simulink model "full_system_forDispatch_lut"  (R2015b)
settings: Solver=VariableStepAuto  StartTime=0.0  StopTime=7  FixedStep=1  RelTol=1e-2
values from neighbouring files (symbols this model uses):
  G1 = 12    [Parameters.m]
  G2 = 50    [Parameters.m]
  Kt = .07329    (= 0.07329)    [Parameters.m]
  L = 1e-4/2    (= 5e-05)    [Parameters.m]
  N = 4    [Parameters.m]
  r = 11*.0254/2    (= 0.1397)    [Parameters.m]
undefined symbols (not defined in the file or in its folder): ad, aq, bd, bq, c_drag_pro, cd, cq, DiscIntNeverNeededParam, dynamic, F_N, Ki, Kp, magnitude, n1, n2, sigbuilder_block, static, T, third_phase, viscous
libraries: fl_lib x24, nesl_utility x16, simulink x3, pe_lib x2
settings Model: Creator=Martin Andersen  LastModifiedBy=Martin Andersen
settings SolverCC: AlgebraicLoopSolver=LineSearch

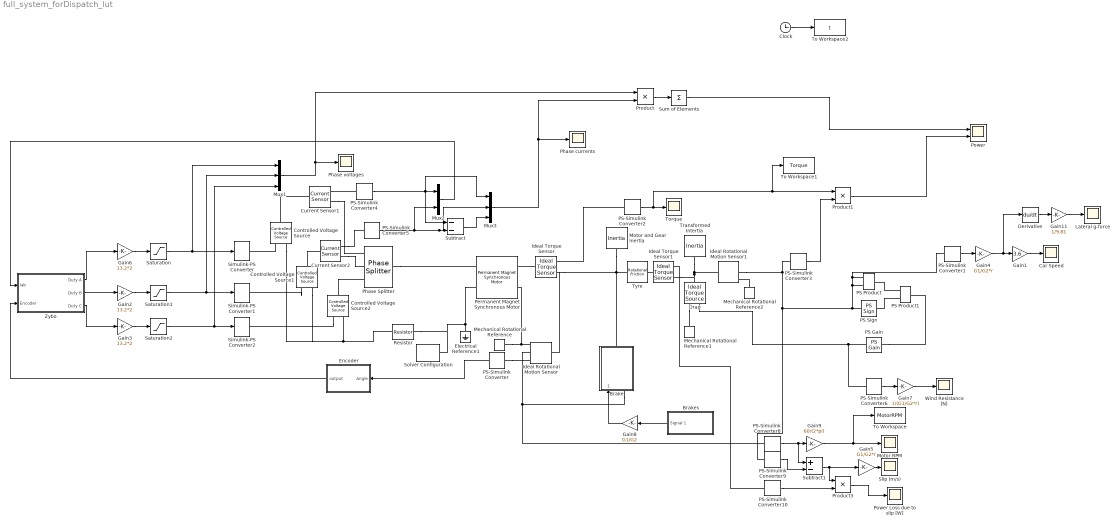
== system full_system_forDispatch_lut ==
  Brake : Subsystem
  Brakes : Subsystem  Tag=STV Subsys  LoadFcn=sigbuilder_block('load');  StartFcn=sigbuilder_block('start');  StopFcn=sigbuilder_block('stop');  ClipboardFcn=sigbuilder_block('clipboard');  mask(Sigbuilder block){}
      mask help: Simulink:masks:SigbuilderBlock_MD
      mask init:
      | if ~strcmp(get_param(bdroot(gcbh),'SimulationStatus'),'stopped') tuvar = sigbuilder_block('maskInit'); end
      settings: CopyFcn=sigbuilder_block('copy');  DeleteFcn=sigbuilder_block('delete');  ModelCloseFcn=sigbuilder_block('modelClose');  PreSaveFcn=sigbuilder_block('preSave');  PauseFcn=sigbuilder_block('pause');  ContinueFcn=sigbuilder_block('continue');  NameChangeFcn=sigbuilder_block('namechange');  OpenFcn=sigbuilder_block('open',[437.6 199.2 550.4 400 ]);  CloseFcn=sigbuilder_block('close');
      mask Display: plot(0, 0, 100, 100,[2, 2, 32, 32, 2], [68, 8, 8, 68, 68],[32, 2], [38, 38], [32, 19, 2],[53, 60, 44], [32, 17, 17, 2],[16, 16, 31, 31]);txt = getActiveGroup(gcbh);text(2, 100, txt,'verticalAlignment', 'top');
  Car Speed : Scope
  Clock : Clock
  Controlled Voltage Source : fl_lib/Electrical/Electrical Sources/Controlled Voltage Source
  Controlled Voltage Source1 : fl_lib/Electrical/Electrical Sources/Controlled Voltage Source
  Controlled Voltage Source2 : fl_lib/Electrical/Electrical Sources/Controlled Voltage Source
  Current Sensor1 : fl_lib/Electrical/Electrical Sensors/Current Sensor
  Current Sensor2 : fl_lib/Electrical/Electrical Sensors/Current Sensor
  Derivative : Derivative
  Drag : fl_lib/Mechanical/Mechanical Sources/Ideal Torque Source
  Electrical Reference1 : fl_lib/Electrical/Electrical Elements/Electrical Reference
  Encoder : Subsystem
  Gain1 : Gain  Gain=3.6
  Gain11 : Gain  Gain=1/9.81
  Gain2 : Gain  Gain=13.2*2
  Gain3 : Gain  Gain=13.2*2
  Gain4 : Gain  Gain=G1/G2*r
  Gain5 : Gain  Gain=G1/G2*r
  Gain6 : Gain  Gain=13.2*2
  Gain7 : Gain  Gain=1/(G1/G2*r)
  Gain8 : Gain  Gain=G1/G2
  Gain9 : Gain  Gain=60/(2*pi)
  Ideal Rotational Motion Sensor : fl_lib/Mechanical/Mechanical Sensors/Ideal Rotational Motion Sensor  offset=0 rad
  Ideal Rotational Motion Sensor1 : fl_lib/Mechanical/Mechanical Sensors/Ideal Rotational Motion Sensor  offset=0 rad
  Ideal Torque Sensor : fl_lib/Mechanical/Mechanical Sensors/Ideal Torque Sensor
  Ideal Torque Sensor1 : fl_lib/Mechanical/Mechanical Sensors/Ideal Torque Sensor
  Lateral g-force : Scope
  Mechanical Rotational Reference : fl_lib/Mechanical/Rotational Elements/Mechanical Rotational Reference
  Mechanical Rotational Reference1 : fl_lib/Mechanical/Rotational Elements/Mechanical Rotational Reference
  Mechanical Rotational Reference2 : fl_lib/Mechanical/Rotational Elements/Mechanical Rotational Reference
  Motor RPM : Scope
  Motor and Gear inertia : fl_lib/Mechanical/Rotational Elements/Inertia  inertia=J_pro1 kg*m^2  w_specify=off  w_priority=None  w=0 rad/s  t_specify=off  t_priority=None  t=0 N*m
  Mux1 : Mux  Inputs=3
  Mux2 : Mux  Inputs=2
  Mux3 : Mux  Inputs=3
  PS Gain : fl_lib/Physical Signals/Functions/PS Gain  gain=c_drag_pro
  PS Product : fl_lib/Physical Signals/Functions/PS Product
  PS Product1 : fl_lib/Physical Signals/Functions/PS Product
  PS Sign : fl_lib/Physical Signals/Nonlinear Operators/PS Sign
  PS-Simulink Converter{,1..6,8..10} (10 alike) : nesl_utility/PS-Simulink Converter  PhysicalDomain=network_engine_domain  SubClassName=ps_output  LeftPortType=input  RightPortType=output  PseudoPeriodic=off  Frequencies=[]  Unit=1  AffineConversion=off
  Permanent Magnet Synchronous Motor : pe_lib/Machines/Permanent Magnet Rotor/Permanent Magnet Synchronous Motor  nPolePairs=N  pm_flux_linkage=Kt/N Wb  stator_param=1  Ld=L H  Lq=L H  L0=L H  Ls=L H  Lm=0 H  Ms=L/10 H  Rs=R Ohm  initial_currents=[0, 0, 0] A  axes_param=2  angular_position0=0 rad  rotor_offset=- pi / 2 rad  shift_3ph=[nan, nan, nan] rad  sqrt2OverSqrt3=nan  oneOverSqrt2=nan  twoPiOver3=nan  Lmin=1e-9 H
  Phase Splitter : pe_lib/Connections/Phase Splitter
  Phase currents : Scope
  Phase voltages : Scope
  Power : Scope  NumInputPorts=2
  Power Loss due to slip [W] : Scope
  Product : Product
  Product1 : Product
  Product3 : Product
  Resistor : fl_lib/Electrical/Electrical Elements/Resistor  R=1e9 Ohm  i_specify=off  i_priority=None  i=0 A  v_specify=off  v_priority=None  v=0 V
  Saturation : Saturate  UpperLimit=13.2*2  LowerLimit=-13.2*2
  Saturation1 : Saturate  UpperLimit=13.2*2  LowerLimit=-13.2*2
  Saturation2 : Saturate  UpperLimit=13.2*2  LowerLimit=-13.2*2
  Simulink-PS Converter : nesl_utility/Simulink-PS Converter  PhysicalDomain=network_engine_domain  SubClassName=ps_input  LeftPortType=input  RightPortType=output  PseudoPeriodic=off  Frequencies=[]  NoiseDistribution=none  NoiseParameters=[]  Unit=1  AffineConversion=off  InputFiltering=off  SimscapeFilterOrder=1  InputFilterTimeConstant=0.001  UdotUserProvided=1
  Simulink-PS Converter1 : nesl_utility/Simulink-PS Converter  PhysicalDomain=network_engine_domain  SubClassName=ps_input  LeftPortType=input  RightPortType=output  PseudoPeriodic=off  Frequencies=[]  NoiseDistribution=none  NoiseParameters=[]  Unit=1  AffineConversion=off  InputFiltering=off  SimscapeFilterOrder=1  InputFilterTimeConstant=0.001  UdotUserProvided=1
  Simulink-PS Converter2 : nesl_utility/Simulink-PS Converter  PhysicalDomain=network_engine_domain  SubClassName=ps_input  LeftPortType=input  RightPortType=output  PseudoPeriodic=off  Frequencies=[]  NoiseDistribution=none  NoiseParameters=[]  Unit=1  AffineConversion=off  InputFiltering=off  SimscapeFilterOrder=1  InputFilterTimeConstant=0.001  UdotUserProvided=1
  Slip (m/s) : Scope
  Solver Configuration : nesl_utility/Solver Configuration  PhysicalDomain=network_engine_domain  SubClassName=solver  LeftPortType=input  RightPortType=generic  Accelerate=off  Tones=[]  Harmonics=[]  SimulateNoise=off  Profile=off  UseLocalSampling=off  EnableSwitchedLinearOptims=on  FrequencyDomain=off  UseCCode=off  RelTol=0.001  AbsTol=1e-06  MinStep=1e-09  ToWorkspace=off  RevertToSquareIcSolve=off  NumHomotopyIterations=100  PhasorMode=off  PhasorModeNumHarmonics=1  DoDC=off  ResidualTolerance=1e-09  UseLocalSolver=off  LocalSolverChoice=NE_BACKWARD_EULER_ADVANCER  LocalSolverSampleTime=0.001  DoFixedCost=off  MaxNonlinIter=3  MaxModeIter=2  LinearAlgebra=Sparse  DelaysMemoryBudget=1024  AutomaticFiltering=on  FilteringTimeConstant=0.001
  Subtract : Sum  Inputs=--
  Subtract1 : Sum  Inputs=+-
  Sum of Elements : Sum  Inputs=+
  To Workspace : ToWorkspace  VariableName=MotorRPM  SampleTime=-1
  To Workspace1 : ToWorkspace  VariableName=Torque  SampleTime=-1
  To Workspace2 : ToWorkspace  VariableName=t  SampleTime=-1
  Torque : Scope
  Transformed Intertia : fl_lib/Mechanical/Rotational Elements/Inertia  inertia=J_pro2 kg*m^2  w_specify=off  w_priority=None  w=0 rad/s  t_specify=off  t_priority=None  t=0 N*m
  Tyre : fl_lib/Mechanical/Rotational Elements/Rotational Friction  brkwy_trq=F_N*static*r*G1/G2 N*m  Col_trq=F_N*dynamic*r*G1/G2 N*m  visc_coef=F_N*viscous*r*G1/G2 N*m/(rad/s)  trans_coef=10 s/rad  vel_thr=1e-4 rad/s  w_specify=off  w_priority=None  w=0 rad/s  t_specify=off  t_priority=None  t=0 N*m
  Wind Resistance [N] : Scope
  Zybo : Subsystem
  wires:
  Gain1/1 -> Car Speed/1
  PS-Simulink Converter4/1 -> Subtract/1, Mux3/1, Mux2/1
  PS-Simulink Converter5/1 -> Mux3/2, Subtract/2, Mux2/2
  PS-Simulink Converter6/1 -> Gain7/1
  Mux1/1 -> Product/1, Phase voltages/1
  Mux2/1 -> Zybo/1(Iab)
  Product/1 -> Sum of Elements/1
  PS-Simulink Converter3/1 -> Product1/2
  Zybo/1(Duty A) -> Gain6/1
  PS-Simulink Converter/1 -> Encoder/1(Angle)
  Encoder/1(output) -> Zybo/2(Encoder)
  Gain6/1 -> Saturation/1
  Gain2/1 -> Saturation1/1
  Gain3/1 -> Saturation2/1
  Saturation/1 -> Mux1/1, Simulink-PS Converter/1
  Saturation1/1 -> Mux1/2, Simulink-PS Converter1/1
  Zybo/2(Duty B) -> Gain2/1
  Zybo/3(Duty C) -> Gain3/1
  Saturation2/1 -> Mux1/3, Simulink-PS Converter2/1
  Subtract/1 -> Mux3/3
  Mux3/1 -> Phase currents/1, Product/2
  Product1/1 -> Power/2
  Brakes/1(Signal 1) -> Gain8/1
  Gain7/1 -> Wind Resistance [N]/1
  PS-Simulink Converter9/1 -> Subtract1/2
  Subtract1/1 -> Product3/1, Gain5/1
  Gain5/1 -> Slip (m/s)/1
  PS-Simulink Converter8/1 -> Subtract1/1, Gain9/1
  PS-Simulink Converter10/1 -> Product3/2
  Gain9/1 -> To Workspace/1, Motor RPM/1
  PS-Simulink Converter2/1 -> To Workspace1/1, Product1/1, Torque/1
  Product3/1 -> Power Loss due to slip [W]/1
  PS-Simulink Converter1/1 -> Gain4/1
  Derivative/1 -> Gain11/1
  Gain11/1 -> Lateral g-force/1
  Gain8/1 -> Brake/1(Brake torque)
  Sum of Elements/1 -> Power/1
  Gain4/1 -> Derivative/1, Gain1/1
  Clock/1 -> To Workspace2/1
  connections:
  Permanent Magnet Synchronous Motor/LConn2 -- Solver Configuration/RConn1 -- Resistor/RConn1 -- Electrical Reference1/LConn1
  Ideal Rotational Motion Sensor/RConn1 -- Mechanical Rotational Reference/LConn1 -- Permanent Magnet Synchronous Motor/RConn2
  PS-Simulink Converter3/LConn1 -- Ideal Rotational Motion Sensor1/RConn2 -- PS-Simulink Converter9/LConn1 -- PS Sign/LConn1 -- PS-Simulink Converter1/LConn1 -- PS Product/LConn1 -- PS Product/LConn2
  PS Product1/LConn2 -- PS Sign/RConn1
  PS Product1/LConn1 -- PS Product/RConn1
  PS Gain/LConn1 -- PS Product1/RConn1
  PS-Simulink Converter6/LConn1 -- Drag/RConn1 -- PS Gain/RConn1
  PS-Simulink Converter/LConn1 -- Ideal Rotational Motion Sensor/RConn3
  Controlled Voltage Source/RConn1 -- Simulink-PS Converter/RConn1
  Controlled Voltage Source1/RConn1 -- Simulink-PS Converter1/RConn1
  Controlled Voltage Source2/RConn1 -- Simulink-PS Converter2/RConn1
  Controlled Voltage Source2/LConn1 -- Phase Splitter/RConn3
  Controlled Voltage Source1/RConn2 -- Controlled Voltage Source/RConn2 -- Resistor/LConn1 -- Controlled Voltage Source2/RConn2
  Phase Splitter/LConn1 -- Permanent Magnet Synchronous Motor/LConn1
  Current Sensor1/LConn1 -- Controlled Voltage Source/LConn1
  Current Sensor1/RConn2 -- Phase Splitter/RConn1
  Current Sensor2/LConn1 -- Controlled Voltage Source1/LConn1
  Current Sensor2/RConn2 -- Phase Splitter/RConn2
  PS-Simulink Converter4/LConn1 -- Current Sensor1/RConn1
  Current Sensor2/RConn1 -- PS-Simulink Converter5/LConn1
  Drag/RConn2 -- Mechanical Rotational Reference1/LConn1
  Ideal Rotational Motion Sensor/LConn1 -- Ideal Torque Sensor/RConn1 -- Brake/RConn1 -- Motor and Gear inertia/LConn1 -- Tyre/LConn1
  PS-Simulink Converter2/LConn1 -- Ideal Torque Sensor/RConn2
  Ideal Torque Sensor/LConn1 -- Permanent Magnet Synchronous Motor/RConn1
  Drag/LConn1 -- Ideal Torque Sensor1/RConn1 -- Ideal Rotational Motion Sensor1/LConn1 -- Transformed Intertia/LConn1
  Mechanical Rotational Reference2/LConn1 -- Ideal Rotational Motion Sensor1/RConn1
  PS-Simulink Converter8/LConn1 -- Ideal Rotational Motion Sensor/RConn2 -- Brake/LConn1
  Tyre/RConn1 -- Ideal Torque Sensor1/LConn1
  PS-Simulink Converter10/LConn1 -- Ideal Torque Sensor1/RConn2

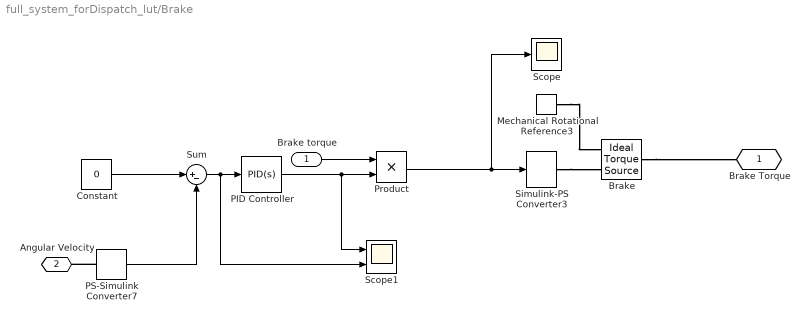
== system full_system_forDispatch_lut/Brake ==
  Brake torque : Inport
  Brake : fl_lib/Mechanical/Mechanical Sources/Ideal Torque Source
  Constant : Constant  Value=0
  Mechanical Rotational Reference3 : fl_lib/Mechanical/Rotational Elements/Mechanical Rotational Reference
  PID Controller : simulink/Continuous/PID Controller  Controller=PID  TimeDomain=Continuous-time  SampleTime=-1  IntegratorMethod=Forward Euler  FilterMethod=Forward Euler  Form=Parallel  UseFilter=on  ControllerParametersSource=internal  P=100  I=50000  D=-.1  N=100  InitialConditionSource=internal  InitialConditionForIntegrator=0  InitialConditionForFilter=0  ExternalReset=none  LimitOutput=on  UpperSaturationLimit=1  LowerSaturationLimit=-1  LinearizeAsGain=on  AntiWindupMode=back-calculation  Kb=100000  TrackingMode=off  Kt=1  PParamMin=[]  PParamMax=[]  IParamMin=[]  IParamMax=[]  DParamMin=[]  DParamMax=[]  NParamMin=[]  NParamMax=[]  KbParamMin=[]  KbParamMax=[]  KtParamMin=[]  KtParamMax=[]  POutMin=[]  POutMax=[]  IOutMin=[]  IOutMax=[]  DOutMin=[]  DOutMax=[]  NOutMin=[]  NOutMax=[]  KbOutMin=[]  KbOutMax=[]  KtOutMin=[]  KtOutMax=[]  IntegratorOutMin=[]  IntegratorOutMax=[]  FilterOutMin=[]  FilterOutMax=[]  SumOutMin=[]  SumOutMax=[]  SumI1OutMin=[]  SumI1OutMax=[]  SumI2OutMin=[]  SumI2OutMax=[]  SumI3OutMin=[]  SumI3OutMax=[]  SumDOutMin=[]  SumDOutMax=[]  SaturationOutMin=[]  SaturationOutMax=[]  IntegratorContinuousStateAttributes=''  IntegratorStateMustResolveToSignalObject=off  IntegratorRTWStateStorageClass=Auto  FilterContinuousStateAttributes=''  FilterStateMustResolveToSignalObject=off  FilterRTWStateStorageClass=Auto  DifferentiatorICPrevScaledInput=0  DifferentiatorOutMin=[]  DifferentiatorOutMax=[]
  PS-Simulink Converter7 : nesl_utility/PS-Simulink Converter  PhysicalDomain=network_engine_domain  SubClassName=ps_output  LeftPortType=input  RightPortType=output  PseudoPeriodic=off  Frequencies=[]  Unit=1  AffineConversion=off
  Product : Product
  Scope : Scope
  Scope1 : Scope  NumInputPorts=2
  Simulink-PS Converter3 : nesl_utility/Simulink-PS Converter  PhysicalDomain=network_engine_domain  SubClassName=ps_input  LeftPortType=input  RightPortType=output  PseudoPeriodic=off  Frequencies=[]  NoiseDistribution=none  NoiseParameters=[]  Unit=1  AffineConversion=off  InputFiltering=off  SimscapeFilterOrder=1  InputFilterTimeConstant=0.001  UdotUserProvided=1
  Sum : Sum  Inputs=|+-
  Brake Torque : PMIOPort  Port=1  Side=Right
  Angular Velocity : PMIOPort  Port=2  Side=Left
  wires:
  Product/1 -> Scope/1, Simulink-PS Converter3/1
  Sum/1 -> Scope1/2, PID Controller/1
  PID Controller/1 -> Scope1/1, Product/2
  Brake torque/1 -> Product/1
  Constant/1 -> Sum/1
  PS-Simulink Converter7/1 -> Sum/2
  connections:
  PS-Simulink Converter7/LConn1 -- Angular Velocity/RConn1
  Brake/LConn1 -- Brake Torque/RConn1
  Mechanical Rotational Reference3/LConn1 -- Brake/RConn2
  Simulink-PS Converter3/RConn1 -- Brake/RConn1

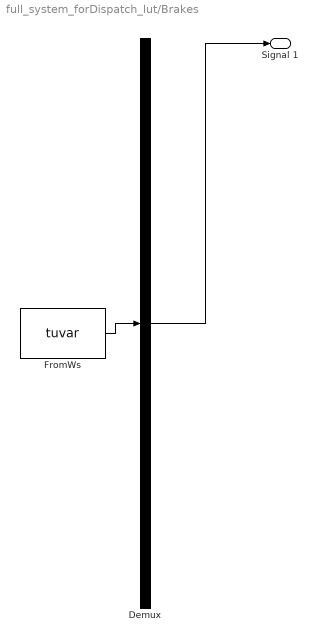
== system full_system_forDispatch_lut/Brakes ==
  Demux : Demux  Tag=STV Demux  Outputs=1
  FromWs : FromWorkspace  Tag=STV FromWs  VariableName=tuvar  SampleTime=0
      SigBuilderData=|
      | common.afterFinalStr = 'Extrapolate'
      | common.sampleTime = 0
      | dataSet.timeRange = [0 10]
      | dataSet.name = 'Group 1'
      | sbobj.Groups.Name = 'Group 1'
      | sbobj.Groups.Signals.Name = 'Signal 1'
      | sbobj.Groups.Signals.XData = [0 5.18 5.34 6.34 6.5 10]
      | sbobj.Groups.Signals.YData = [0 0 100 188.5 0 0]
  Signal 1 : Outport  Tag=STV Outport
  wires:
  Demux/1 -> Signal 1/1
  FromWs/1 -> Demux/1

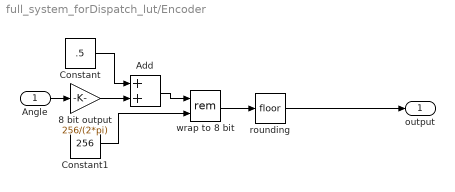
== system full_system_forDispatch_lut/Encoder ==
  Angle : Inport
  8 bit output : Gain  Gain=256/(2*pi)
  Add : Sum
  Constant : Constant  Value=.5
  Constant1 : Constant  Value=256
  rounding : Rounding
  wrap to 8 bit : Math  Operator=rem  SaturateOnIntegerOverflow=on
  output : Outport
  wires:
  wrap to 8 bit/1 -> rounding/1
  Constant1/1 -> wrap to 8 bit/2
  Angle/1 -> 8 bit output/1
  rounding/1 -> output/1
  8 bit output/1 -> Add/2
  Add/1 -> wrap to 8 bit/1
  Constant/1 -> Add/1

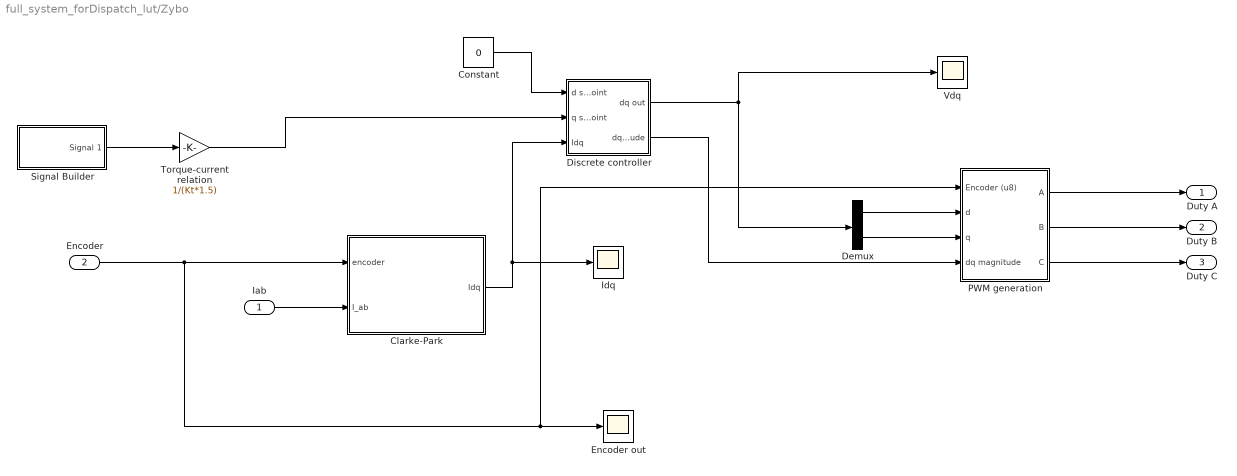
== system full_system_forDispatch_lut/Zybo ==
  Iab : Inport
  Encoder : Inport  Port=2
  Clarke-Park : Subsystem  SystemSampleTime=T
  Constant : Constant  Value=0
  Demux : Demux  Outputs=2
  Discrete controller : Subsystem  TreatAsAtomicUnit=on  SystemSampleTime=T
  Encoder out : Scope
  Idq : Scope
  PWM generation : Subsystem
  Signal Builder : Subsystem  Tag=STV Subsys  LoadFcn=sigbuilder_block('load');  StartFcn=sigbuilder_block('start');  StopFcn=sigbuilder_block('stop');  ClipboardFcn=sigbuilder_block('clipboard');  mask(Sigbuilder block){}
      mask help: Simulink:masks:SigbuilderBlock_MD
      mask init:
      | if ~strcmp(get_param(bdroot(gcbh),'SimulationStatus'),'stopped') tuvar = sigbuilder_block('maskInit'); end
      settings: CopyFcn=sigbuilder_block('copy');  DeleteFcn=sigbuilder_block('delete');  ModelCloseFcn=sigbuilder_block('modelClose');  PreSaveFcn=sigbuilder_block('preSave');  PauseFcn=sigbuilder_block('pause');  ContinueFcn=sigbuilder_block('continue');  NameChangeFcn=sigbuilder_block('namechange');  OpenFcn=sigbuilder_block('open',[298.8 170.4 550.8 400.2 ]);  CloseFcn=sigbuilder_block('close');
      mask Display: plot(0, 0, 100, 100,[2, 2, 32, 32, 2], [68, 8, 8, 68, 68],[32, 2], [38, 38], [32, 19, 2],[53, 60, 44], [32, 17, 17, 2],[16, 16, 31, 31]);txt = getActiveGroup(gcbh);text(2, 100, txt,'verticalAlignment', 'top');
  Torque-current relation : Gain  Gain=1/(Kt*1.5)
  Vdq : Scope
  Duty A : Outport
  Duty B : Outport  Port=2
  Duty C : Outport  Port=3
  wires:
  Demux/1 -> PWM generation/2(d)
  Discrete controller/2(dq magnitude) -> PWM generation/4(dq magnitude)
  Demux/2 -> PWM generation/3(q)
  PWM generation/3(C) -> Duty C/1
  PWM generation/1(A) -> Duty A/1
  PWM generation/2(B) -> Duty B/1
  Torque-current relation/1 -> Discrete controller/2(q setpoint)
  Signal Builder/1(Signal 1) -> Torque-current relation/1
  Discrete controller/1(dq out) -> Vdq/1, Demux/1
  Iab/1 -> Clarke-Park/2(I_ab)
  Clarke-Park/1(Idq) -> Idq/1, Discrete controller/3(Idq)
  Encoder/1 -> Clarke-Park/1(encoder), PWM generation/1(Encoder (u8)), Encoder out/1
  Constant/1 -> Discrete controller/1(d setpoint)

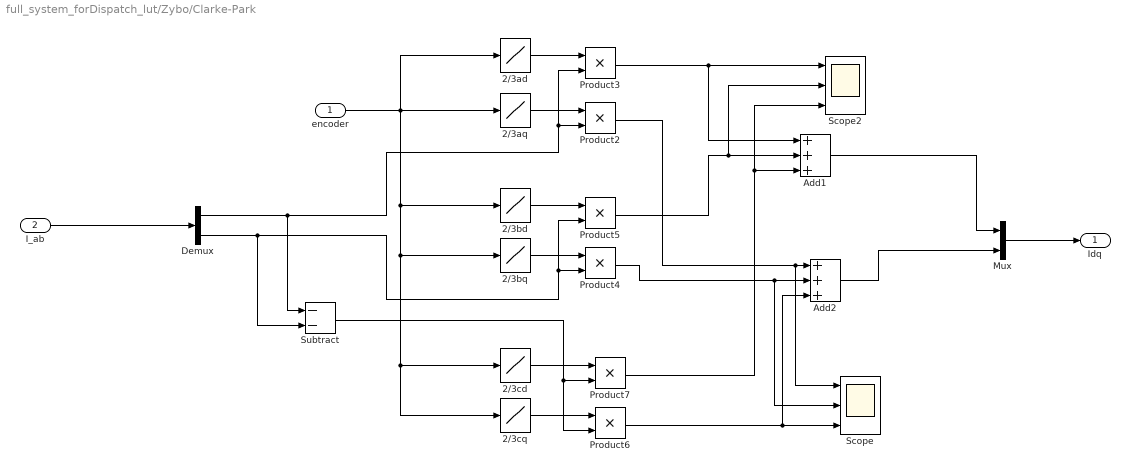
== system full_system_forDispatch_lut/Zybo/Clarke-Park ==
  encoder : Inport
  I_ab : Inport  Port=2
  2/3ad : Lookup_n-D  NumberOfTableDimensions=1  BreakpointsForDimension1=n1  Table=ad*2/3  InterpMethod=Nearest  InternalRulePriority=Speed  RndMeth=Simplest  InputSameDT=on
  2/3aq : Lookup_n-D  NumberOfTableDimensions=1  BreakpointsForDimension1=n1  Table=aq*2/3  InterpMethod=Nearest  InternalRulePriority=Speed  RndMeth=Simplest  InputSameDT=on
  2/3bd : Lookup_n-D  NumberOfTableDimensions=1  BreakpointsForDimension1=n1  Table=bd*2/3  InterpMethod=Nearest  InternalRulePriority=Speed  RndMeth=Simplest  InputSameDT=on
  2/3bq : Lookup_n-D  NumberOfTableDimensions=1  BreakpointsForDimension1=n1  Table=bq*2/3  InterpMethod=Nearest  InternalRulePriority=Speed  RndMeth=Simplest  InputSameDT=on
  2/3cd : Lookup_n-D  NumberOfTableDimensions=1  BreakpointsForDimension1=n1  Table=cd*2/3  InterpMethod=Nearest  InternalRulePriority=Speed  RndMeth=Simplest  InputSameDT=on
  2/3cq : Lookup_n-D  NumberOfTableDimensions=1  BreakpointsForDimension1=n1  Table=cq*2/3  InterpMethod=Nearest  InternalRulePriority=Speed  RndMeth=Simplest  InputSameDT=on
  Add1 : Sum  Inputs=+++
  Add2 : Sum  Inputs=+++
  Demux : Demux  Outputs=2
  Mux : Mux  Inputs=2
  Product{2..7} (6 alike) : Product
  Scope : Scope  NumInputPorts=3
  Scope2 : Scope  NumInputPorts=3
  Subtract : Sum  Inputs=--
  Idq : Outport
  wires:
  Add2/1 -> Mux/2
  2/3ad/1 -> Product3/1
  2/3cq/1 -> Product6/1
  Demux/1 -> Product2/2, Product3/2, Subtract/1
  2/3bq/1 -> Product4/1
  I_ab/1 -> Demux/1
  Subtract/1 -> Product6/2, Product7/2
  Product6/1 -> Scope/3, Add2/3
  Product4/1 -> Scope/2, Add2/2
  2/3aq/1 -> Product2/1
  Product5/1 -> Scope2/2, Add1/2
  2/3bd/1 -> Product5/1
  Demux/2 -> Subtract/2, Product5/2, Product4/2
  2/3cd/1 -> Product7/1
  Product3/1 -> Scope2/1, Add1/1
  Product2/1 -> Scope/1, Add2/1
  Product7/1 -> Scope2/3, Add1/3
  encoder/1 -> 2/3cq/1, 2/3cd/1, 2/3bq/1, 2/3bd/1, 2/3aq/1, 2/3ad/1
  Mux/1 -> Idq/1
  Add1/1 -> Mux/1

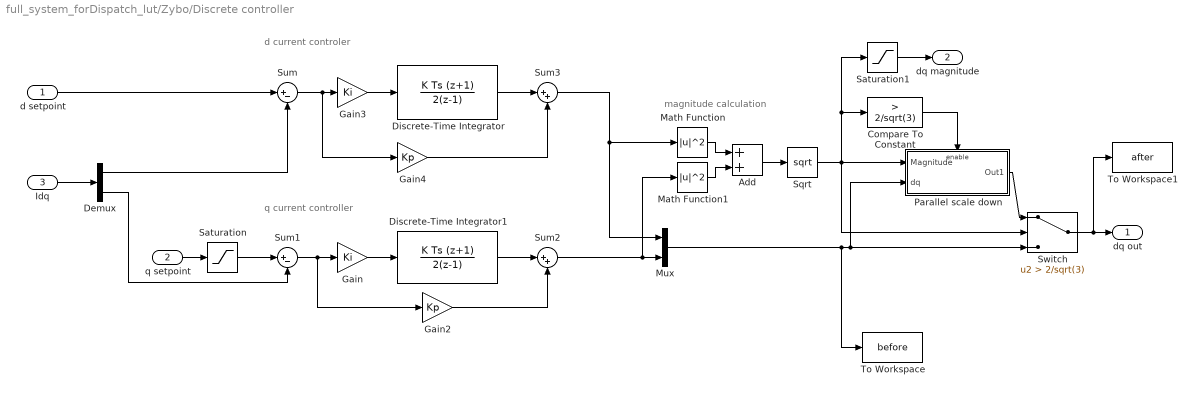
== system full_system_forDispatch_lut/Zybo/Discrete controller ==
  note: magnitude calculation
  note: d current controler
  note: q current controller
  d setpoint : Inport
  q setpoint : Inport  Port=2
  Idq : Inport  Port=3
  Add : Sum
  Compare To Constant : simulink/Logic and Bit Operations/Compare To Constant  relop=>  const=2/sqrt(3)  OutDataTypeStr=boolean
  Demux : Demux  Outputs=2
  Discrete-Time Integrator : DiscreteIntegrator  IntegratorMethod=Integration: Trapezoidal  InitialConditionSetting=State (most efficient)  SampleTime=T  LimitOutput=on  UpperSaturationLimit=2/sqrt(3)  LowerSaturationLimit=-2/sqrt(3)  ICPrevOutput=DiscIntNeverNeededParam  ICPrevScaledInput=DiscIntNeverNeededParam
  Discrete-Time Integrator1 : DiscreteIntegrator  IntegratorMethod=Integration: Trapezoidal  InitialConditionSetting=State (most efficient)  SampleTime=T  LimitOutput=on  UpperSaturationLimit=2/sqrt(3)  LowerSaturationLimit=-2/sqrt(3)  ICPrevOutput=DiscIntNeverNeededParam  ICPrevScaledInput=DiscIntNeverNeededParam
  Gain : Gain  Gain=Ki
  Gain2 : Gain  Gain=Kp
  Gain3 : Gain  Gain=Ki
  Gain4 : Gain  Gain=Kp
  Math Function : Math  Operator=magnitude^2  SaturateOnIntegerOverflow=on
  Math Function1 : Math  Operator=magnitude^2  SaturateOnIntegerOverflow=on
  Mux : Mux  Inputs=2
  Parallel scale down : Subsystem  TreatAsAtomicUnit=on
  Saturation : Saturate  UpperLimit=300
  Saturation1 : Saturate  UpperLimit=2/sqrt(3)
  Sqrt : Sqrt  SaturateOnIntegerOverflow=on
  Sum : Sum  Inputs=|+-
  Sum1 : Sum  Inputs=|+-
  Sum2 : Sum  Inputs=|++
  Sum3 : Sum  Inputs=|++
  Switch : Switch  Criteria=u2 > Threshold  Threshold=2/sqrt(3)
  To Workspace : ToWorkspace  VariableName=before  SampleTime=-1
      settings: Save2DSignal=2-D array (concatenate along first dimension)
  To Workspace1 : ToWorkspace  VariableName=after  SampleTime=-1
      settings: Save2DSignal=2-D array (concatenate along first dimension)
  dq out : Outport
  dq magnitude : Outport  Port=2
  wires:
  Gain4/1 -> Sum3/2
  Sum/1 -> Gain4/1, Gain3/1
  Gain2/1 -> Sum2/2
  Gain/1 -> Discrete-Time Integrator1/1
  Gain3/1 -> Discrete-Time Integrator/1
  Discrete-Time Integrator/1 -> Sum3/1
  Mux/1 -> To Workspace/1, Switch/3, Parallel scale down/2(dq)
  Sum3/1 -> Mux/1, Math Function/1
  Sum2/1 -> Mux/2, Math Function1/1
  Math Function/1 -> Add/1
  Math Function1/1 -> Add/2
  Add/1 -> Sqrt/1
  q setpoint/1 -> Saturation/1
  d setpoint/1 -> Sum/1
  Saturation/1 -> Sum1/1
  Switch/1 -> To Workspace1/1, dq out/1
  Compare To Constant/1 -> Parallel scale down/Enable
  Parallel scale down/1(Out1) -> Switch/1
  Sqrt/1 -> Compare To Constant/1, Saturation1/1, Parallel scale down/1(Magnitude), Switch/2
  Idq/1 -> Demux/1
  Saturation1/1 -> dq magnitude/1
  Sum1/1 -> Gain2/1, Gain/1
  Discrete-Time Integrator1/1 -> Sum2/1
  Demux/2 -> Sum1/2
  Demux/1 -> Sum/2

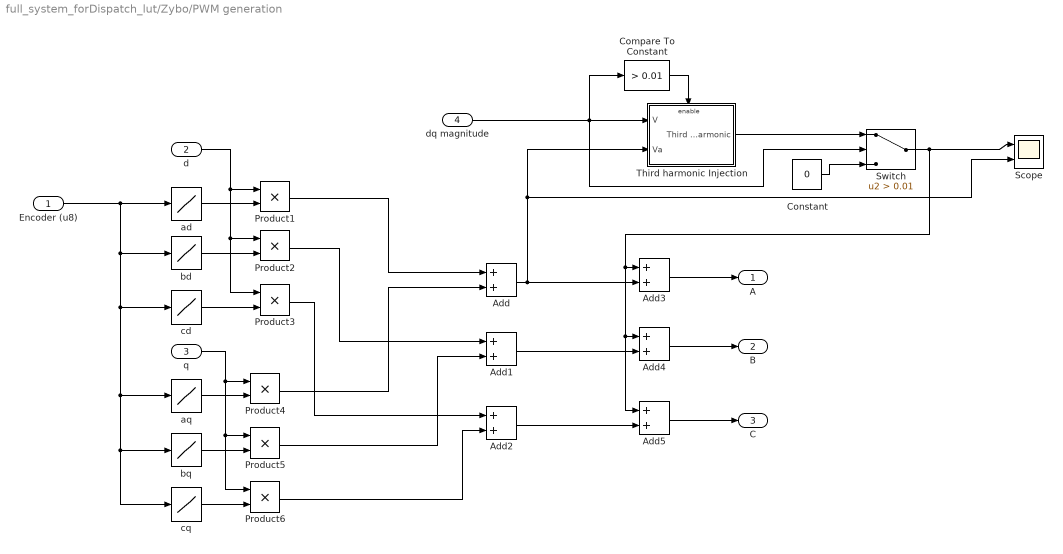
== system full_system_forDispatch_lut/Zybo/PWM generation ==
  Encoder (u8) : Inport
  d : Inport  Port=2
  q : Inport  Port=3
  dq magnitude : Inport  Port=4
  Add{,1..5} (6 alike) : Sum
  Compare To Constant : simulink/Logic and Bit Operations/Compare To Constant  relop=>  const=0.01  OutDataTypeStr=boolean
  Constant : Constant  Value=0
  Product{1..6} (6 alike) : Product
  Scope : Scope  NumInputPorts=2
  Switch : Switch  Criteria=u2 > Threshold  Threshold=0.01
  Third harmonic Injection : Subsystem
  ad : Lookup_n-D  NumberOfTableDimensions=1  BreakpointsForDimension1=n1  IndexSearchMethod=Linear search  Table=ad  InterpMethod=Nearest  InternalRulePriority=Speed  RndMeth=Simplest  InputSameDT=on
  aq : Lookup_n-D  NumberOfTableDimensions=1  BreakpointsForDimension1=n1  Table=aq  InterpMethod=Nearest  InternalRulePriority=Speed  RndMeth=Simplest  InputSameDT=on
  bd : Lookup_n-D  NumberOfTableDimensions=1  BreakpointsForDimension1=n1  Table=bd  InterpMethod=Nearest  InternalRulePriority=Speed  RndMeth=Simplest  InputSameDT=on
  bq : Lookup_n-D  NumberOfTableDimensions=1  BreakpointsForDimension1=n1  Table=bq  InterpMethod=Nearest  InternalRulePriority=Speed  RndMeth=Simplest  InputSameDT=on
  cd : Lookup_n-D  NumberOfTableDimensions=1  BreakpointsForDimension1=n1  Table=cd  InterpMethod=Nearest  InternalRulePriority=Speed  RndMeth=Simplest  InputSameDT=on
  cq : Lookup_n-D  NumberOfTableDimensions=1  BreakpointsForDimension1=n1  Table=cq  InterpMethod=Nearest  InternalRulePriority=Speed  RndMeth=Simplest  InputSameDT=on
  A : Outport
  B : Outport  Port=2
  C : Outport  Port=3
  wires:
  Encoder (u8)/1 -> cq/1, bq/1, aq/1, cd/1, bd/1, ad/1
  cd/1 -> Product3/2
  bd/1 -> Product2/2
  ad/1 -> Product1/2
  d/1 -> Product3/1, Product2/1, Product1/1
  bq/1 -> Product5/2
  cq/1 -> Product6/2
  aq/1 -> Product4/2
  q/1 -> Product6/1, Product5/1, Product4/1
  Add5/1 -> C/1
  Add4/1 -> B/1
  Add3/1 -> A/1
  Add1/1 -> Add4/2
  Add/1 -> Scope/2, Third harmonic Injection/2(Va), Add3/2
  Add2/1 -> Add5/2
  Product1/1 -> Add/1
  Product4/1 -> Add/2
  Product2/1 -> Add1/1
  Product5/1 -> Add1/2
  Product3/1 -> Add2/1
  Product6/1 -> Add2/2
  dq magnitude/1 -> Switch/2, Compare To Constant/1, Third harmonic Injection/1(V)
  Switch/1 -> Scope/1, Add5/1, Add4/1, Add3/1
  Third harmonic Injection/1(Third Harmonic) -> Switch/1
  Compare To Constant/1 -> Third harmonic Injection/Enable
  Constant/1 -> Switch/3

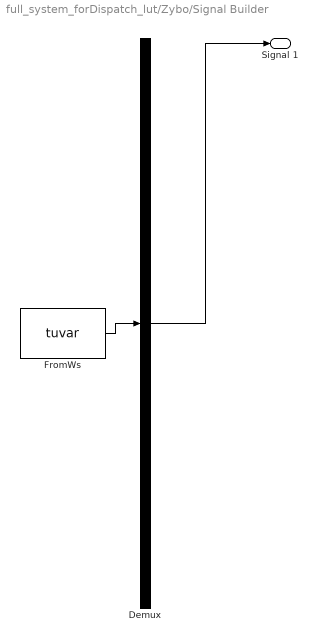
== system full_system_forDispatch_lut/Zybo/Signal Builder ==
  Demux : Demux  Tag=STV Demux  Outputs=1
  FromWs : FromWorkspace  Tag=STV FromWs  VariableName=tuvar  SampleTime=0
      SigBuilderData=|
      | common.afterFinalStr = 'Extrapolate'
      | common.sampleTime = 0
      | dataSet.timeRange = [0 10]
      | dataSet.name = 'Group 1'
      | sbobj.Groups.Name = 'Group 1'
      | sbobj.Groups.Signals.Name = 'Signal 1'
      | sbobj.Groups.Signals.XData = [0 0.32 5.02 5.02 6.64 6.64 10]
      | sbobj.Groups.Signals.YData = [0 40 40.4 -0.2 0 20.2 25]
  Signal 1 : Outport  Tag=STV Outport
  wires:
  Demux/1 -> Signal 1/1
  FromWs/1 -> Demux/1

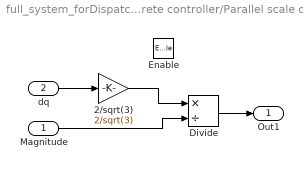
== system full_system_forDispatch_lut/Zybo/Discrete controller/Parallel scale down ==
  Magnitude : Inport
  dq : Inport  Port=2
  Enable : EnablePort
  2/sqrt(3) : Gain  Gain=2/sqrt(3)
  Divide : Product  Inputs=*/
  Out1 : Outport
  wires:
  dq/1 -> 2/sqrt(3)/1
  Magnitude/1 -> Divide/2
  Divide/1 -> Out1/1
  2/sqrt(3)/1 -> Divide/1

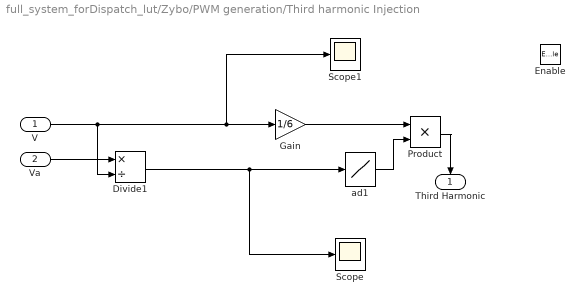
== system full_system_forDispatch_lut/Zybo/PWM generation/Third harmonic Injection ==
  V : Inport
  Va : Inport  Port=2
  Enable : EnablePort
  Divide1 : Product  Inputs=*/
  Gain : Gain  Gain=1/6
  Product : Product
  Scope : Scope
  Scope1 : Scope
  ad1 : Lookup_n-D  NumberOfTableDimensions=1  BreakpointsForDimension1=n2  Table=third_phase  InterpMethod=Nearest  InternalRulePriority=Speed  RndMeth=Simplest  InputSameDT=on
  Third Harmonic : Outport
  wires:
  V/1 -> Divide1/2, Scope1/1, Gain/1
  Gain/1 -> Product/1
  ad1/1 -> Product/2
  Product/1 -> Third Harmonic/1
  Va/1 -> Divide1/1
  Divide1/1 -> Scope/1, ad1/1
